simulink model "Zad1_model_22b"  (R2022b)
settings: Solver=ode4  StartTime=0.0  StopTime=8  FixedStep=0.001  RelTol=1e-3
values from neighbouring files (symbols this model uses):
  A = [0 1; -6 -5]    [Zad1.m]
  B = [0; 6]    [Zad1.m]
  C = [1 0]    [Zad1.m]
  D = 0    [Zad1.m]
  h = h_max/20    (= 0.10471975512)    [Zad1.m]
undefined symbols (not defined in the file or in its folder): A_discr, B_discr, C_discr, D_discr, freq, x0
settings Model: Creator=dz2yk3  LastModifiedBy=janro

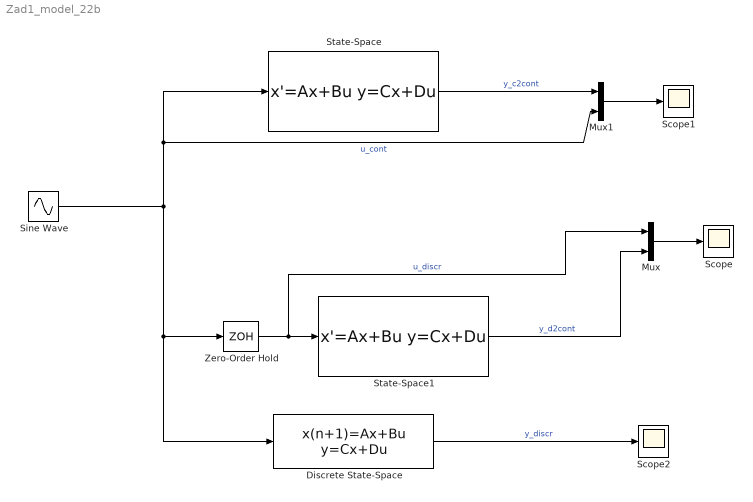
== system Zad1_model_22b ==
  Discrete State-Space : DiscreteStateSpace  A=A_discr  B=B_discr  C=C_discr  D=D_discr  InitialCondition=x0  SampleTime=round(h,3)
  Mux : Mux  Inputs=2
  Mux1 : Mux  Inputs=2
  Scope : Scope
  Scope1 : Scope
  Scope2 : Scope
  Sine Wave : Sin  Bias=1  Frequency=freq  SampleTime=0
  State-Space : StateSpace  A=A  B=B  C=C  D=D  InitialCondition=x0
  State-Space1 : StateSpace  A=A  B=B  C=C  D=D  InitialCondition=x0
  Zero-Order Hold : ZeroOrderHold  SampleTime=round(h,3)
  wires:
  Mux/1 -> Scope/1
  State-Space/1 -> Mux1/1  "y_c2cont"
  Sine Wave/1 -> Discrete State-Space/1, Zero-Order Hold/1, Mux1/2, State-Space/1  "u_cont"
  Zero-Order Hold/1 -> Mux/1, State-Space1/1  "u_discr"
  State-Space1/1 -> Mux/2  "y_d2cont"
  Mux1/1 -> Scope1/1
  Discrete State-Space/1 -> Scope2/1  "y_discr"
